simulink model "uz_pmsm_model_2022b"  (R2022b)
settings: Solver=FixedStepAuto  StartTime=0.0  StopTime=0.05  RelTol=1e-3
PreLoadFcn:
  | uz_pmsm_model_init_parameter
PostLoadFcn:
  | % Import the data from Excel for a lookup table
  | FluxMapData = readtable('C:\Users\Philipp\ultrazohm\ultrazohm_sw\ip_cores\uz_pmsm_model\FluxMapData_2023-05-26_13-07-57.csv');
  | % Row indices for lookup table
  | d_current_in_d_axis = FluxMapData(8:27,1:end);
  | % Column indices for lookup table
  | q_current_in_d_axis = FluxMapData(29:48,1:end);
  | % Output values for lookup table
  | d_Flux_d_axis = FluxMapData(50:69,1:end);
values from neighbouring files (symbols this model uses):
  ad1 = ad_1(1)    [LUT_approx_methode2a.m]    (also in LUT_approx_methode2a_clean.m = ad_self(1); LUT_approx_methode_2a_FEM.m; fitting_parameter.mat = 0.03048394862; fitting_parameter_48V_SynRM.mat = 0.0218446789236)
  ad2 = ad_1(2)    [LUT_approx_methode2a.m]    (also in LUT_approx_methode2a_clean.m = ad_self(2); LUT_approx_methode_2a_FEM.m; fitting_parameter.mat = 0.0402440194669; fitting_parameter_48V_SynRM.mat = 0.015691946268)
  ad3 = ad_1(3)    [LUT_approx_methode2a.m]    (also in LUT_approx_methode2a_clean.m = ad_self(3); LUT_approx_methode_2a_FEM.m; fitting_parameter.mat = -16.4812001193; fitting_parameter_48V_SynRM.mat = 2.77465564774)
  ad4 = ad_3_6(1)    [LUT_approx_methode2a.m]    (also in LUT_approx_methode2a_clean.m = ad_4_6(1); LUT_approx_methode_2a_FEM.m; fitting_parameter.mat = 1.2964378241; fitting_parameter_48V_SynRM.mat = 0.0214529395212)
  ad5 = ad_3_6(2)    [LUT_approx_methode2a.m]    (also in LUT_approx_methode2a_clean.m = ad_4_6(2); LUT_approx_methode_2a_FEM.m; fitting_parameter.mat = 0.000618316734858; fitting_parameter_48V_SynRM.mat = 0.0128514742508)
  ad6 = ad_3_6(3)    [LUT_approx_methode2a.m]    (also in LUT_approx_methode2a_clean.m = ad_4_6(3); LUT_approx_methode_2a_FEM.m; fitting_parameter.mat = -12.2755860444; fitting_parameter_48V_SynRM.mat = 2.54408267654)
  aq1 = aq_1(1)    [LUT_approx_methode2a.m]    (also in LUT_approx_methode2a_clean.m = aq_self(1); LUT_approx_methode_2a_FEM.m; fitting_parameter.mat = 0.0048166705291; fitting_parameter_48V_SynRM.mat = 0.00205546577039)
  aq2 = aq_1(2)    [LUT_approx_methode2a.m]    (also in LUT_approx_methode2a_clean.m = aq_self(2); LUT_approx_methode_2a_FEM.m; fitting_parameter.mat = 0.171595255564; fitting_parameter_48V_SynRM.mat = 0.0602932843871)
  aq3 = aq_1(3)    [LUT_approx_methode2a.m]    (also in LUT_approx_methode2a_clean.m = aq_self(3); LUT_approx_methode_2a_FEM.m; fitting_parameter.mat = 0.000926293864031; fitting_parameter_48V_SynRM.mat = 4.42738872822e-05)
  aq4 = aq_3_6(1)    [LUT_approx_methode2a.m]    (also in LUT_approx_methode2a_clean.m = aq_4_6(1); LUT_approx_methode_2a_FEM.m; fitting_parameter.mat = 0.00500187099075; fitting_parameter_48V_SynRM.mat = 0.000698420875152)
  aq5 = aq_3_6(2)    [LUT_approx_methode2a.m]    (also in LUT_approx_methode2a_clean.m = aq_4_6(2); LUT_approx_methode_2a_FEM.m; fitting_parameter.mat = 0.17052123489; fitting_parameter_48V_SynRM.mat = 0.0493122483219)
  aq6 = aq_3_6(3)    [LUT_approx_methode2a.m]    (also in LUT_approx_methode2a_clean.m = aq_4_6(3); LUT_approx_methode_2a_FEM.m; fitting_parameter.mat = 0.00091860845; fitting_parameter_48V_SynRM.mat = 4.14644316065e-05)
  d_current_d_Flux = FluxMapData{1,1:20}    [uz_pmsm_model_init_parameter.m]
  d_current_q_Flux = FluxMapData{66,1:20}    [uz_pmsm_model_init_parameter.m]
  entkopplung_dynamic = false    [compare_simulation_to_measurement.m]    (also in uz_pmsm_model_init_parameter.m; uz_pmsm_model_init_parameter_clean.m)
  entkopplung_linear = true    [compare_simulation_to_measurement.m]    (also in uz_pmsm_model_init_parameter.m; uz_pmsm_model_init_parameter_clean.m = false)
  entkopplung_static = false    [compare_simulation_to_measurement.m]    (also in uz_pmsm_model_init_parameter.m; uz_pmsm_model_init_parameter_clean.m)
  Fid1_Giq1 = ((1/2).*(aq3-aq6).*((q_current_set).^2))+((aq1./aq2).*log(cosh(aq2.*q_current_set)))-((aq4/aq5).*log(cosh(aq5.*q_current_set)))    [LUT_approx_methode2a.m]    (also in LUT_approx_methode2a_clean.m; LUT_approx_methode_2a_FEM.m = (1/2).*(aq3-aq6).*((q_current_set).^2)+((aq1./aq2).*log(cosh; fitting_parameter.mat = -0.00135679401385; fitting_parameter_48V_SynRM.mat = 0.221350145237)
  Fid2_Giq2 = ((ad1./ad2).*(log(cosh(ad2.*(d_current_set-ad3))))) - ((ad4./ad5).*(log(cosh(ad5.*(d_current_set-ad6)))))    [LUT_approx_methode2a.m]    (also in LUT_approx_methode2a_clean.m; LUT_approx_methode_2a_FEM.m = ((ad1./ad2).*(log(cosh(ad2.*(d_current_set-ad3))))) - (((ad1; fitting_parameter.mat = 0.0788137932988; fitting_parameter_48V_SynRM.mat = 0.221214979406)
  Flux_d = FluxMapData{43:62,1:20}'*(1e-3)    [uz_pmsm_model_init_parameter.m]
  Flux_q = FluxMapData{108:127,1:20}'*(1e-3)    [uz_pmsm_model_init_parameter.m]
  friction_coefficient = 0.001    [uz_pmsm_model_init_parameter.m]    (also in uz_pmsm_model_init_parameter_clean.m)
  inertia = 0.000084    (= 8.4e-05)    [uz_pmsm_model_init_parameter.m]    (also in uz_pmsm_model_init_parameter_clean.m)
  L_d = 0.00045    [uz_pmsm_model_init_parameter.m]    (also in uz_pmsm_model_init_parameter_clean.m)
  L_q = 0.002    [uz_pmsm_model_init_parameter.m]    (also in uz_pmsm_model_init_parameter_clean.m)
  parameter_nachfuerung = false    [compare_simulation_to_measurement.m]    (also in uz_pmsm_model_init_parameter.m; uz_pmsm_model_init_parameter_clean.m)
  polepair = 4    [uz_pmsm_model_init_parameter.m]    (also in uz_pmsm_model_init_parameter_clean.m)
  praediktion_entkopplung_nonlinear = false    [compare_simulation_to_measurement.m]    (also in uz_pmsm_model_init_parameter.m; uz_pmsm_model_init_parameter_clean.m = true)
  psi_pm = 0.0194    [uz_pmsm_model_init_parameter.m]    (also in uz_pmsm_model_init_parameter_clean.m)
  q_current_d_Flux = FluxMapData{22:41,1}    [uz_pmsm_model_init_parameter.m]
  q_current_q_Flux = FluxMapData{87:106,1}    [uz_pmsm_model_init_parameter.m]
  R_1 = 0.3    [uz_pmsm_model_init_parameter.m]    (also in uz_pmsm_model_init_parameter_clean.m)
  simulate_mechanical = true    [compare_simulation_to_measurement.m]    (also in export_csv.m = false; uz_pmsm_model_init_parameter.m = false; uz_pmsm_model_init_parameter_clean.m = false)
  simulate_nonlinear_modell = false    [compare_simulation_to_measurement.m]    (also in uz_pmsm_model_init_parameter.m = true; uz_pmsm_model_init_parameter_clean.m = true)
  simulate_open_loop = true    [compare_simulation_to_measurement.m]    (also in export_csv.m; uz_pmsm_model_init_parameter.m = false; uz_pmsm_model_init_parameter_clean.m = false)
  static_friction_torque = 0.01    [uz_pmsm_model_init_parameter.m]    (also in uz_pmsm_model_init_parameter_clean.m)
  tau_sum = 2*ts_regler    (= 0.0001)    [uz_pmsm_model_init_parameter.m]    (also in uz_pmsm_model_init_parameter_clean.m = 8e-05)
  ts = logs{k}.Values    [export_csv.m]    (also in uz_pmsm_model_init_parameter.m = 2e-06; uz_pmsm_model_init_parameter_clean.m = 2e-06)
  ts_regler = 1/20e3    (= 5e-05)    [uz_pmsm_model_init_parameter.m]    (also in uz_pmsm_model_init_parameter_clean.m = 4e-05)
undefined symbols (not defined in the file or in its folder): Ki_Bo_d, Ki_Bo_q, Kp_Bo_d, Kp_Bo_q, Ldq
libraries: slpidlib x6
(part 1 of 4)
settings Model: DataTypeOverride=Off  NumberOfSteps=100  Creator=ts  LastModifiedBy=Philipp
settings SolverCC: AlgebraicLoopSolver=TrustRegion  AutoInsertRateTranBlk=on
settings DataIOCC: LimitDataPoints=on  SaveOutput=off  SaveTime=off
settings OptimizationCC: BlockReduction=off  ConditionallyExecuteInputs=off  DefaultParameterBehavior=Inlined  DefaultUnderspecifiedDataType=single  ReuseModelBlockBuffer=on  LifeSpan=inf
settings DebuggingCC: AlgebraicLoopMsg=error  SingleTaskRateTransMsg=error  UnconnectedInputMsg=warning  UnconnectedOutputMsg=warning  UnconnectedLineMsg=warning  AllowSymbolicDim=off  StrictBusMsg=ErrorOnBusTreatedAsVector  SFUnexpectedBacktrackingDiag=warning  SFNoUnconditionalDefaultTransitionDiag=warning  SFExecutionAtInitializationDiag=none  ArithmeticOperatorsInVariantConditions=warning
settings HardwareCC: ProdBitPerPointer=32  ProdBitPerSizeT=32  ProdBitPerPtrDiffT=32  ProdLargestAtomicFloat=None  ProdIntDivRoundTo=Undefined  ProdEndianess=Unspecified  ProdWordSize=32  ProdHWDeviceType=ASIC/FPGA->ASIC/FPGA  ProdEqTarget=off
settings ModelReferenceCC: EnableRefExpFcnMdlSchedulingChecks=on
settings SFSimCC: SimUseLocalCustomCode=off  CustomCodeUndefinedFunction=UseInterfaceOnly
settings RTWCC: RTWUseLocalCustomCode=off  DLArmComputeVersion=19.05
settings CodeAppCC: StateflowObjectComments=on
settings GRTTargetCC: TargetLangStandard=C89/C90 (ANSI)
settings ConfigComp: CovScope=ReferencedModels  CovMetricSettings=dw  CovSaveCumulativeToWorkspaceVar=on  CovSaveSingleToWorkspaceVar=on  CovExternalEMLEnable=off  CovSFcnEnable=off

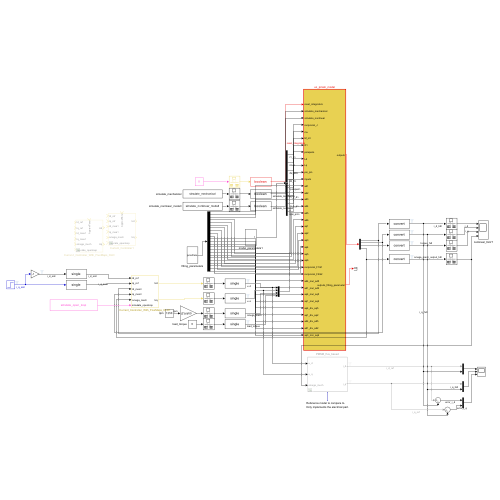
[thumbnail: Simulink's stored preview of the top-level diagram]
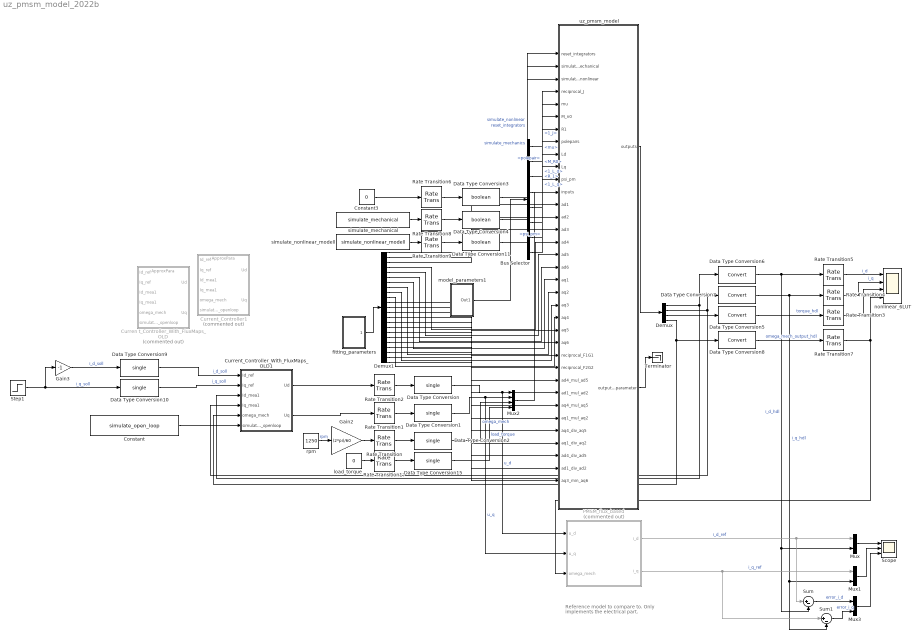
== system uz_pmsm_model_2022b ==
  note: Reference model to compare to.
      | Only implements the electrical part.
  Bus Selector : BusSelector  OutputSignals=1_J,mu,M_R0,R_1,polepair,1_L_d,1_L_q,psi_pm
  Constant : Constant  Value=simulate_open_loop
  Constant3 : Constant  Value=0
  Curren t_Controller_With_FluxMaps_OLD : Subsystem  Commented=on
      settings: PortSchema="{\"entries\":[{\"content\":{\"sides\":[{\"content\":{\"connectorIds\":[\"In1\",\"In2\",\"In3\",\"In4\",\"In5\",\"In6\"]},\"type\":\"ConnectorPlacement.EquallySpacedRectSide\",\"uuid\":\"af970c43-a604-4c86-9598-367deed13f4b\"},{\"content\":{\"connectorIds\":[\"Out1\",\"Out2\"],\"side\":\"RIGHT\"},\"type\":\"ConnectorPlacement.EquallySpacedRectSide\",\"uuid\":\"dab3805d-2102-4aac-8fbd-bf5dcc1227bc\"},{\"content\":{\"connectorIds\":[\"In7\"],\"side\":\"TOP\"},\"type\":\"ConnectorPlacement.EquallySpacedRectSide\",\"uuid\":\"2748ff21-16e6-4765-af5f-5654ece797e9\"}]},\"type\":\"ConnectorPlacement.EquallySpacedConnector\",\"uuid\":\"76312914-9df7-46a3-b8a6-6bdd22bb9fc1\"}],\"packageUris\":[\"http://schema.mathworks.com/mf0/Connector/R2020b\"],\"version\":\"1.0\"}"
  Current_Controller1 : Subsystem  Commented=on
      settings: PortSchema="{\"entries\":[{\"content\":{\"sides\":[{\"content\":{\"connectorIds\":[\"In1\",\"In2\",\"In3\",\"In4\",\"In5\",\"In6\"]},\"type\":\"ConnectorPlacement.EquallySpacedRectSide\",\"uuid\":\"af970c43-a604-4c86-9598-367deed13f4b\"},{\"content\":{\"connectorIds\":[\"Out1\",\"Out2\"],\"side\":\"RIGHT\"},\"type\":\"ConnectorPlacement.EquallySpacedRectSide\",\"uuid\":\"dab3805d-2102-4aac-8fbd-bf5dcc1227bc\"},{\"content\":{\"connectorIds\":[\"In7\"],\"side\":\"TOP\"},\"type\":\"ConnectorPlacement.EquallySpacedRectSide\",\"uuid\":\"2748ff21-16e6-4765-af5f-5654ece797e9\"}]},\"type\":\"ConnectorPlacement.EquallySpacedConnector\",\"uuid\":\"76312914-9df7-46a3-b8a6-6bdd22bb9fc1\"}],\"packageUris\":[\"http://schema.mathworks.com/mf0/Connector/R2020b\"],\"version\":\"1.0\"}"
  Current_Controller_With_FluxMaps_OLD1 : Subsystem
  Data Type Conversion{,1..2,9..10,15} (6 alike) : DataTypeConversion  OutDataTypeStr=single  SaturateOnIntegerOverflow=off  RndMeth=Floor
  Data Type Conversion11 : DataTypeConversion  OutDataTypeStr=boolean  SaturateOnIntegerOverflow=off  RndMeth=Floor
  Data Type Conversion3 : DataTypeConversion  OutDataTypeStr=boolean  SaturateOnIntegerOverflow=off  RndMeth=Floor
  Data Type Conversion4 : DataTypeConversion  OutDataTypeStr=boolean  SaturateOnIntegerOverflow=off  RndMeth=Floor
  Data Type Conversion{5..8} (4 alike) : DataTypeConversion  SaturateOnIntegerOverflow=off  RndMeth=Floor
  Demux : Demux
  Demux1 : Demux  Outputs=23
  Gain2 : Gain  Gain=(2*pi)/60
  Gain3 : Gain  Gain=-1
  Mux : Mux  Inputs=2
  Mux1 : Mux  Inputs=2
  Mux2 : Mux
  Mux3 : Mux  Inputs=2
  PMSM_flux_based : Subsystem  Commented=on
  Rate Transition{,1..2,6,8..9,17} (7 alike) : RateTransition  OutPortSampleTime=ts
  Rate Transition{3..5,7} (4 alike) : RateTransition
  Scope : Scope  NumInputPorts=3
  Step1 : Step  Time=0.025  After=10
  Sum : Sum  Inputs=|+-
  Sum1 : Sum  Inputs=|+-
  Terminator : Terminator
  fitting_parameters : Subsystem
  load_torque : Constant  Value=0
  model_parameters1 : Subsystem
  nonlinear_6LUT : Scope  NumInputPorts=4
  rpm : Constant  Value=1250
  simulate_mechanical : Constant  Value=simulate_mechanical
  simulate_nonlinear_modell : Constant  Value=simulate_nonlinear_modell
  uz_pmsm_model : Subsystem  TreatAsAtomicUnit=on
  wires:
  Rate Transition/1 -> Data Type Conversion2/1
  Rate Transition1/1 -> Data Type Conversion1/1
  Rate Transition2/1 -> Data Type Conversion/1
  Data Type Conversion6/1 -> Mux/2, Sum/2, Rate Transition5/1  "i_d_hdl"
  Data Type Conversion7/1 -> Rate Transition4/1, Mux1/2, Sum1/2  "i_q_hdl"
  Data Type Conversion5/1 -> Rate Transition3/1  "torque_hdl"
  Rate Transition4/1 -> nonlinear_6LUT/2  "i_q"
  Rate Transition5/1 -> nonlinear_6LUT/1  "i_d"
  Rate Transition3/1 -> nonlinear_6LUT/3
  Rate Transition6/1 -> Data Type Conversion3/1
  Constant3/1 -> Rate Transition6/1
  Rate Transition8/1 -> Data Type Conversion4/1
  simulate_mechanical/1 -> Rate Transition8/1
  Data Type Conversion3/1 -> uz_pmsm_model/1(reset_integrators)  "reset_integrators"
  Data Type Conversion4/1 -> uz_pmsm_model/2(simulate_mechanical)  "simulate_mechanics"
  load_torque/1 -> Rate Transition17/1
  Rate Transition17/1 -> Data Type Conversion15/1
  Mux/1 -> Scope/1
  Mux1/1 -> Scope/2
  PMSM_flux_based/2(i_q) -> Mux1/1, Sum1/1  "i_q_ref"
  PMSM_flux_based/1(i_d) -> Mux/1, Sum/1  "i_d_ref"
  Data Type Conversion8/1 -> Rate Transition7/1  "omega_mech_output_hdl"
  Rate Transition7/1 -> PMSM_flux_based/3(omega_mech), nonlinear_6LUT/4
  Bus Selector/1 -> uz_pmsm_model/4(reciprocal_J)  "<1_J>"
  Bus Selector/2 -> uz_pmsm_model/5(mu)  "<mu>"
  Bus Selector/3 -> uz_pmsm_model/6(M_n0)  "<M_R0>"
  Bus Selector/4 -> uz_pmsm_model/7(R1)  "<R_1>"
  Bus Selector/5 -> uz_pmsm_model/8(polepairs)  "<polepair>"
  model_parameters1/1(Out1) -> Bus Selector/1
  Sum/1 -> Mux3/1  "error_i_d"
  Sum1/1 -> Mux3/2  "error_i_q"
  Mux3/1 -> Scope/3
  Step1/1 -> Gain3/1, Data Type Conversion10/1  "i_q_soll"
  Demux/3 -> Data Type Conversion5/1
  Gain3/1 -> Data Type Conversion9/1  "i_d_soll"
  Demux/1 -> Current_Controller_With_FluxMaps_OLD1/3(Id_mea1), Data Type Conversion6/1
  Demux/4 -> Current_Controller_With_FluxMaps_OLD1/5(omega_mech), Data Type Conversion8/1
  Demux/2 -> Data Type Conversion7/1, Current_Controller_With_FluxMaps_OLD1/4(Iq_mea1)
  Data Type Conversion/1 -> PMSM_flux_based/1(u_d), Mux2/1  "u_d"
  Data Type Conversion1/1 -> PMSM_flux_based/2(u_q), Mux2/2  "u_q"
  Data Type Conversion15/1 -> Mux2/4  "load_torque"
  Data Type Conversion2/1 -> Mux2/3  "omega_mech"
  Mux2/1 -> uz_pmsm_model/12(inputs)
  uz_pmsm_model/1(outputs) -> Demux/1
  Data Type Conversion9/1 -> Current_Controller_With_FluxMaps_OLD1/1(Id_ref)  "i_d_soll"
  Data Type Conversion10/1 -> Current_Controller_With_FluxMaps_OLD1/2(Iq_ref)  "i_q_soll"
  Current_Controller_With_FluxMaps_OLD1/1(Ud) -> Rate Transition2/1
  Current_Controller_With_FluxMaps_OLD1/2(Uq) -> Rate Transition1/1
  Gain2/1 -> Rate Transition/1
  Constant/1 -> Current_Controller_With_FluxMaps_OLD1/6(simulate_openloop)
  rpm/1 -> Gain2/1  "rpm"
  simulate_nonlinear_modell/1 -> Rate Transition9/1
  Rate Transition9/1 -> Data Type Conversion11/1
  Bus Selector/6 -> uz_pmsm_model/9(Ld)  "<1_L_d>"
  Bus Selector/7 -> uz_pmsm_model/10(Lq)  "<1_L_q>"
  Bus Selector/8 -> uz_pmsm_model/11(psi_pm)  "<psi_pm>"
  Data Type Conversion11/1 -> uz_pmsm_model/3(simulate_nonlinear)  "simulate_nonlinear"
  fitting_parameters/1(ApproxPara) -> Demux1/1
  Demux1/1 -> uz_pmsm_model/13(ad1)
  Demux1/2 -> uz_pmsm_model/14(ad2)
  Demux1/3 -> uz_pmsm_model/15(ad3)
  Demux1/4 -> uz_pmsm_model/16(ad4)
  Demux1/5 -> uz_pmsm_model/17(ad5)
  Demux1/6 -> uz_pmsm_model/18(ad6)
  Demux1/7 -> uz_pmsm_model/19(aq1)
  Demux1/8 -> uz_pmsm_model/20(aq2)
  Demux1/9 -> uz_pmsm_model/21(aq3)
  Demux1/10 -> uz_pmsm_model/22(aq4)
  Demux1/11 -> uz_pmsm_model/23(aq5)
  Demux1/12 -> uz_pmsm_model/24(aq6)
  Demux1/13 -> uz_pmsm_model/25(reciprocal_F1G1)
  Demux1/14 -> uz_pmsm_model/26(reciprocal_F2G2)
  Demux1/15 -> uz_pmsm_model/27(ad4_mul_ad5)
  Demux1/16 -> uz_pmsm_model/28(ad1_mul_ad2)
  Demux1/17 -> uz_pmsm_model/29(aq4_mul_aq5)
  Demux1/18 -> uz_pmsm_model/30(aq1_mul_aq2)
  Demux1/19 -> uz_pmsm_model/31(aq4_div_aq5)
  Demux1/20 -> uz_pmsm_model/32(aq1_div_aq2)
  Demux1/21 -> uz_pmsm_model/33(ad4_div_ad5)
  Demux1/22 -> uz_pmsm_model/34(ad1_div_ad2)
  Demux1/23 -> uz_pmsm_model/35(aq3_min_aq6)
  uz_pmsm_model/2(outputs_fitting_parameter) -> Terminator/1

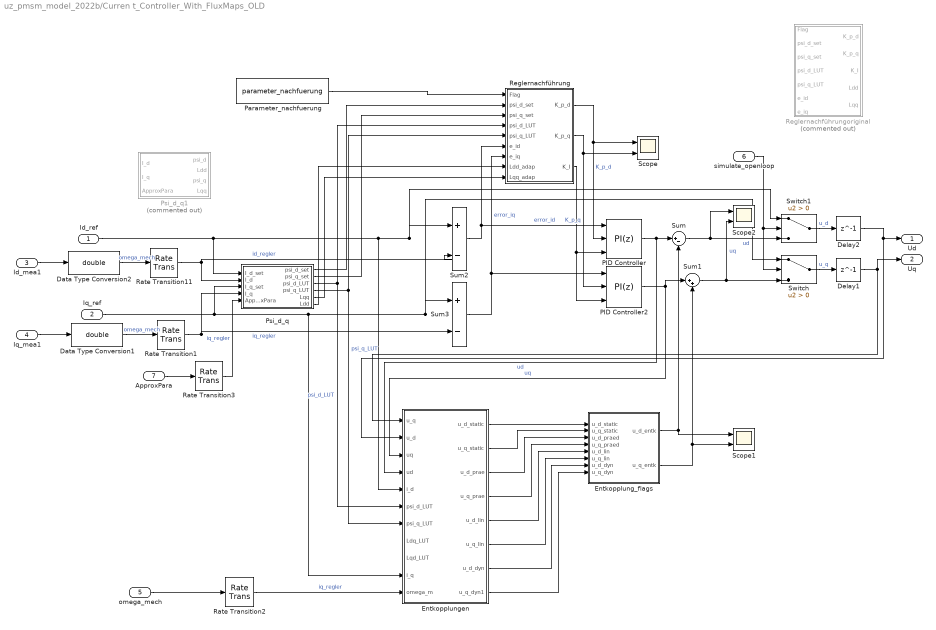
== system uz_pmsm_model_2022b/Curren t_Controller_With_FluxMaps_OLD ==
  Id_ref : Inport
  Iq_ref : Inport  Port=2
  Id_mea1 : Inport  Port=3
  Iq_mea1 : Inport  Port=4
  omega_mech : Inport  Port=5
  simulate_openloop : Inport  Port=6
  ApproxPara : Inport  Port=7
  Data Type Conversion1 : DataTypeConversion  OutDataTypeStr=double  SaturateOnIntegerOverflow=off  RndMeth=Floor
  Data Type Conversion2 : DataTypeConversion  OutDataTypeStr=double  SaturateOnIntegerOverflow=off  RndMeth=Floor
  Delay1 : Delay  DelayLength=1
  Delay2 : Delay  DelayLength=1
  Entkopplung_flags : Subsystem
  Entkopplungen : Subsystem
  PID Controller : slpidlib/PID Controller  Controller=PI  Form=Parallel  TimeDomain=Discrete-time  UseExternalTs=off  SampleTime=-1  IntegratorMethod=Forward Euler  FilterMethod=Forward Euler  ControllerParametersSource=external  P=Kp_Bo_d  I=Ki_Bo_d  UseKiTs=off  D=0  N=100  UseFilter=on  TunerSelectOption=Transfer Function Based (PID Tuner App)  InitialConditionSource=internal  InitialConditionForIntegrator=0  InitialConditionForFilter=0  DifferentiatorICPrevScaledInput=0  ExternalReset=none  TrackingMode=off  Kt=1  LimitOutput=off  SatLimitsSource=internal  UpperSaturationLimit=48  LowerSaturationLimit=-48  LinearizeAsGain=off  AntiWindupMode=clamping  Kb=1  LimitIntegrator=off  UpperIntegratorSaturationLimit=48  LowerIntegratorSaturationLimit=-48  POutMin=[]  POutMax=[]  IOutMin=[]  IOutMax=[]  DOutMin=[]  DOutMax=[]  NOutMin=[]  NOutMax=[]  SumOutMin=[]  SumOutMax=[]  SaturationOutMin=[]  SaturationOutMax=[]  PParamMin=[]  PParamMax=[]  IParamMin=[]  IParamMax=[]  DParamMin=[]  DParamMax=[]  NParamMin=[]  NParamMax=[]  KbParamMin=[]  KbParamMax=[]  KtParamMin=[]  KtParamMax=[]  KbOutMin=[]  KbOutMax=[]  KtOutMin=[]  KtOutMax=[]  IntegratorOutMin=[]  IntegratorOutMax=[]  FilterOutMin=[]  FilterOutMax=[]  SumI1OutMin=[]  SumI1OutMax=[]  SumI2OutMin=[]  SumI2OutMax=[]  SumI3OutMin=[]  SumI3OutMax=[]  SumI4OutMin=[]  SumI4OutMax=[]  SumDOutMin=[]  SumDOutMax=[]  DifferentiatorOutMin=[]  DifferentiatorOutMax=[]  FilterDiffOutCoefMin=[]  FilterDiffOutCoefMax=[]  ReciprocalOutMin=[]  ReciprocalOutMax=[]  SumDenOutMin=[]  SumDenOutMax=[]  SumNumOutMin=[]  SumNumOutMax=[]  DivideOutMin=[]  DivideOutMax=[]  UdiffTsProdOutMin=[]  UdiffTsProdOutMax=[]  NTsProdOutMin=[]  NTsProdOutMax=[]  UintegralTsProdOutMin=[]  UintegralTsProdOutMax=[]  UngainTsProdOutMin=[]  UngainTsProdOutMax=[]  IntegratorContinuousStateAttributes=''  IntegratorStateMustResolveToSignalObject=off  IntegratorRTWStateStorageClass=Auto  FilterContinuousStateAttributes=''  FilterStateMustResolveToSignalObject=off  FilterRTWStateStorageClass=Auto  ParallelPVariant=ExternalParameters  IdealPVariant=Disabled  IVariant=ExternalParameters  DVariant=Disabled  IntegratorVariant=Discrete  SatVariant=Disabled  AWVariant=Passthrough  PCopyVariant=Disabled  TRVariant=Disabled  FdbkBlocksVariant=Forward  IdealPFdbkVariant=Disabled  SatFdbkVariant=Disabled  DerivativeFilterVariant=Disabled  NVariant=Disabled  NCopyVariant=Disabled_SignalSpec  FilterICVariant=Disabled  IntegratorICVariant=InternalICs  ExternalResetVariant=Disabled  TRSumVariant=Passthrough  SumFdbkVariant=Disabled  SumVariant=Sum_PI  TsampFilterVariant=InternalTs  TsampNgainVariant=Passthrough  TsampIntegralVariant=Disabled_SignalSpec  ExternalSaturationOutDataTypeStr=Inherit: Same as second input
  PID Controller2 : slpidlib/PID Controller  Controller=PI  Form=Parallel  TimeDomain=Discrete-time  UseExternalTs=off  SampleTime=-1  IntegratorMethod=Forward Euler  FilterMethod=Forward Euler  ControllerParametersSource=external  P=Kp_Bo_q  I=Ki_Bo_q  UseKiTs=off  D=0  N=100  UseFilter=on  TunerSelectOption=Transfer Function Based (PID Tuner App)  InitialConditionSource=internal  InitialConditionForIntegrator=0  InitialConditionForFilter=0  DifferentiatorICPrevScaledInput=0  ExternalReset=none  TrackingMode=off  Kt=1  LimitOutput=off  SatLimitsSource=internal  UpperSaturationLimit=48  LowerSaturationLimit=-48  LinearizeAsGain=off  AntiWindupMode=clamping  Kb=1  LimitIntegrator=off  UpperIntegratorSaturationLimit=48  LowerIntegratorSaturationLimit=-48  POutMin=[]  POutMax=[]  IOutMin=[]  IOutMax=[]  DOutMin=[]  DOutMax=[]  NOutMin=[]  NOutMax=[]  SumOutMin=[]  SumOutMax=[]  SaturationOutMin=[]  SaturationOutMax=[]  PParamMin=[]  PParamMax=[]  IParamMin=[]  IParamMax=[]  DParamMin=[]  DParamMax=[]  NParamMin=[]  NParamMax=[]  KbParamMin=[]  KbParamMax=[]  KtParamMin=[]  KtParamMax=[]  KbOutMin=[]  KbOutMax=[]  KtOutMin=[]  KtOutMax=[]  IntegratorOutMin=[]  IntegratorOutMax=[]  FilterOutMin=[]  FilterOutMax=[]  SumI1OutMin=[]  SumI1OutMax=[]  SumI2OutMin=[]  SumI2OutMax=[]  SumI3OutMin=[]  SumI3OutMax=[]  SumI4OutMin=[]  SumI4OutMax=[]  SumDOutMin=[]  SumDOutMax=[]  DifferentiatorOutMin=[]  DifferentiatorOutMax=[]  FilterDiffOutCoefMin=[]  FilterDiffOutCoefMax=[]  ReciprocalOutMin=[]  ReciprocalOutMax=[]  SumDenOutMin=[]  SumDenOutMax=[]  SumNumOutMin=[]  SumNumOutMax=[]  DivideOutMin=[]  DivideOutMax=[]  UdiffTsProdOutMin=[]  UdiffTsProdOutMax=[]  NTsProdOutMin=[]  NTsProdOutMax=[]  UintegralTsProdOutMin=[]  UintegralTsProdOutMax=[]  UngainTsProdOutMin=[]  UngainTsProdOutMax=[]  IntegratorContinuousStateAttributes=''  IntegratorStateMustResolveToSignalObject=off  IntegratorRTWStateStorageClass=Auto  FilterContinuousStateAttributes=''  FilterStateMustResolveToSignalObject=off  FilterRTWStateStorageClass=Auto  ParallelPVariant=ExternalParameters  IdealPVariant=Disabled  IVariant=ExternalParameters  DVariant=Disabled  IntegratorVariant=Discrete  SatVariant=Disabled  AWVariant=Passthrough  PCopyVariant=Disabled  TRVariant=Disabled  FdbkBlocksVariant=Forward  IdealPFdbkVariant=Disabled  SatFdbkVariant=Disabled  DerivativeFilterVariant=Disabled  NVariant=Disabled  NCopyVariant=Disabled_SignalSpec  FilterICVariant=Disabled  IntegratorICVariant=InternalICs  ExternalResetVariant=Disabled  TRSumVariant=Passthrough  SumFdbkVariant=Disabled  SumVariant=Sum_PI  TsampFilterVariant=InternalTs  TsampNgainVariant=Passthrough  TsampIntegralVariant=Disabled_SignalSpec  ExternalSaturationOutDataTypeStr=Inherit: Same as second input
  Parameter_nachfuerung : Constant  Value=parameter_nachfuerung
  Psi_d_q : Subsystem
  Psi_d_q1 : Subsystem  Commented=on
  Rate Transition{1..3,11} (4 alike) : RateTransition  OutPortSampleTime=ts_regler
  Reglernachführung : Subsystem
  Reglernachführungoriginal : Subsystem  Commented=on
  Scope : Scope  NumInputPorts=2
  Scope1 : Scope  NumInputPorts=2
  Scope2 : Scope  NumInputPorts=2
  Sum : Sum  Inputs=|+-
  Sum1 : Sum  Inputs=|++
  Sum2 : Sum  Inputs=|+-
  Sum3 : Sum  Inputs=|+-
  Switch : Switch  Criteria=u2 > Threshold  SaturateOnIntegerOverflow=off  InputSameDT=off
  Switch1 : Switch  Criteria=u2 > Threshold  SaturateOnIntegerOverflow=off  InputSameDT=off
  Ud : Outport
  Uq : Outport  Port=2
  wires:
  Sum3/1 -> Reglernachführung/7(e_iq), PID Controller2/1  "error_iq"
  Sum2/1 -> PID Controller/1, Reglernachführung/6(e_id)  "error_id"
  Sum/1 -> Scope2/1, Switch1/3  "ud"
  PID Controller/1 -> Entkopplungen/4(ud), Sum/1  "ud"
  PID Controller2/1 -> Sum1/1, Entkopplungen/3(uq)  "uq"
  Sum1/1 -> Scope2/2, Switch/3  "uq"
  Iq_ref/1 -> Entkopplungen/10(i_q), Sum3/1, Switch/1, Psi_d_q/3(I_q_set)
  Id_ref/1 -> Psi_d_q/1(I_d_set), Entkopplungen/5(i_d), Sum2/1, Switch1/1
  Switch/1 -> Delay1/1  "u_q"
  Switch1/1 -> Delay2/1  "u_d"
  simulate_openloop/1 -> Switch/2, Switch1/2
  Reglernachführung/1(K_p_d) -> PID Controller/2, Scope/1  "K_p_d"
  Reglernachführung/2(K_p_q) -> PID Controller2/2, Scope/2  "K_p_q"
  Reglernachführung/3(K_I) -> PID Controller2/3, PID Controller/3
  Id_mea1/1 -> Data Type Conversion2/1
  Iq_mea1/1 -> Data Type Conversion1/1
  Psi_d_q/3(psi_d_LUT) -> Entkopplungen/6(psi_d_LUT), Reglernachführung/4(psi_d_LUT)  "psi_d_LUT"
  Psi_d_q/4(psi_q_LUT) -> Entkopplungen/7(psi_q_LUT), Reglernachführung/5(psi_q_LUT)  "psi_q_LUT"
  Parameter_nachfuerung/1 -> Reglernachführung/1(Flag)
  Psi_d_q/1(psi_d_set) -> Reglernachführung/2(psi_d_set)
  Psi_d_q/2(psi_q_set) -> Reglernachführung/3(psi_q_set)
  omega_mech/1 -> Rate Transition2/1
  Entkopplungen/1(u_d_static) -> Entkopplung_flags/1(u_d_static)
  Entkopplungen/2(u_q_static) -> Entkopplung_flags/2(u_q_static)
  Entkopplungen/3(u_d_prae) -> Entkopplung_flags/3(u_d_praed)
  Entkopplungen/4(u_q_prae) -> Entkopplung_flags/4(u_q_praed)
  Entkopplungen/5(u_d_lin) -> Entkopplung_flags/5(u_d_lin)
  Entkopplungen/6(u_q_lin) -> Entkopplung_flags/6(u_q_lin)
  Entkopplung_flags/1(u_d_entk) -> Scope1/1, Sum/2
  Entkopplung_flags/2(u_q_entk) -> Scope1/2, Sum1/2
  Rate Transition11/1 -> Sum2/2, Psi_d_q/2(I_d)  "id_regler"
  Rate Transition1/1 -> Sum3/2, Psi_d_q/4(I_q)  "iq_regler"
  Rate Transition2/1 -> Entkopplungen/11(omega_m)  "iq_regler"
  Delay2/1 -> Ud/1, Entkopplungen/2(u_d)
  Delay1/1 -> Uq/1, Entkopplungen/1(u_q)
  Entkopplungen/7(u_d_dyn) -> Entkopplung_flags/7(u_d_dyn)
  Entkopplungen/8(u_q_dyn1) -> Entkopplung_flags/8(u_q_dyn)
  ApproxPara/1 -> Rate Transition3/1
  Rate Transition3/1 -> Psi_d_q/5(ApproxPara)  "iq_regler"
  Data Type Conversion2/1 -> Rate Transition11/1  "omega_mech"
  Data Type Conversion1/1 -> Rate Transition1/1  "omega_mech"
  Psi_d_q/5(Lqq) -> Reglernachführung/9(Lqq_adap)
  Psi_d_q/6(Ldd) -> Reglernachführung/8(Ldd_adap)

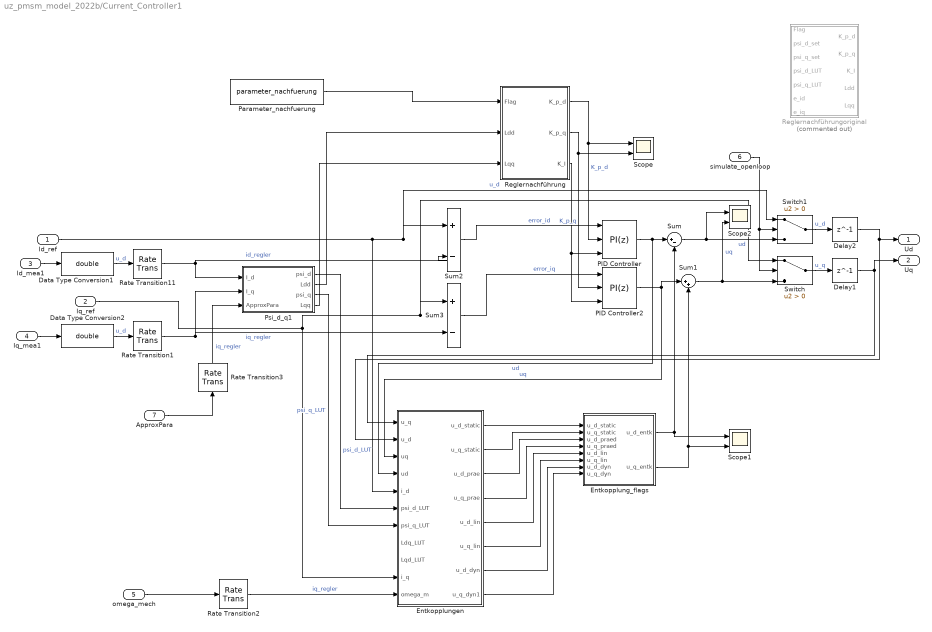
== system uz_pmsm_model_2022b/Current_Controller1 ==
  Id_ref : Inport
  Iq_ref : Inport  Port=2
  Id_mea1 : Inport  Port=3
  Iq_mea1 : Inport  Port=4
  omega_mech : Inport  Port=5
  simulate_openloop : Inport  Port=6
  ApproxPara : Inport  Port=7
  Data Type Conversion1 : DataTypeConversion  OutDataTypeStr=double  SaturateOnIntegerOverflow=off  RndMeth=Floor
  Data Type Conversion2 : DataTypeConversion  OutDataTypeStr=double  SaturateOnIntegerOverflow=off  RndMeth=Floor
  Delay1 : Delay  DelayLength=1
  Delay2 : Delay  DelayLength=1
  Entkopplung_flags : Subsystem
  Entkopplungen : Subsystem
  PID Controller : slpidlib/PID Controller  Controller=PI  Form=Parallel  TimeDomain=Discrete-time  UseExternalTs=off  SampleTime=-1  IntegratorMethod=Forward Euler  FilterMethod=Forward Euler  ControllerParametersSource=external  P=Kp_Bo_d  I=Ki_Bo_d  UseKiTs=off  D=0  N=100  UseFilter=on  TunerSelectOption=Transfer Function Based (PID Tuner App)  InitialConditionSource=internal  InitialConditionForIntegrator=0  InitialConditionForFilter=0  DifferentiatorICPrevScaledInput=0  ExternalReset=none  TrackingMode=off  Kt=1  LimitOutput=off  SatLimitsSource=internal  UpperSaturationLimit=48  LowerSaturationLimit=-48  LinearizeAsGain=off  AntiWindupMode=clamping  Kb=1  LimitIntegrator=off  UpperIntegratorSaturationLimit=48  LowerIntegratorSaturationLimit=-48  POutMin=[]  POutMax=[]  IOutMin=[]  IOutMax=[]  DOutMin=[]  DOutMax=[]  NOutMin=[]  NOutMax=[]  SumOutMin=[]  SumOutMax=[]  SaturationOutMin=[]  SaturationOutMax=[]  PParamMin=[]  PParamMax=[]  IParamMin=[]  IParamMax=[]  DParamMin=[]  DParamMax=[]  NParamMin=[]  NParamMax=[]  KbParamMin=[]  KbParamMax=[]  KtParamMin=[]  KtParamMax=[]  KbOutMin=[]  KbOutMax=[]  KtOutMin=[]  KtOutMax=[]  IntegratorOutMin=[]  IntegratorOutMax=[]  FilterOutMin=[]  FilterOutMax=[]  SumI1OutMin=[]  SumI1OutMax=[]  SumI2OutMin=[]  SumI2OutMax=[]  SumI3OutMin=[]  SumI3OutMax=[]  SumI4OutMin=[]  SumI4OutMax=[]  SumDOutMin=[]  SumDOutMax=[]  DifferentiatorOutMin=[]  DifferentiatorOutMax=[]  FilterDiffOutCoefMin=[]  FilterDiffOutCoefMax=[]  ReciprocalOutMin=[]  ReciprocalOutMax=[]  SumDenOutMin=[]  SumDenOutMax=[]  SumNumOutMin=[]  SumNumOutMax=[]  DivideOutMin=[]  DivideOutMax=[]  UdiffTsProdOutMin=[]  UdiffTsProdOutMax=[]  NTsProdOutMin=[]  NTsProdOutMax=[]  UintegralTsProdOutMin=[]  UintegralTsProdOutMax=[]  UngainTsProdOutMin=[]  UngainTsProdOutMax=[]  IntegratorContinuousStateAttributes=''  IntegratorStateMustResolveToSignalObject=off  IntegratorRTWStateStorageClass=Auto  FilterContinuousStateAttributes=''  FilterStateMustResolveToSignalObject=off  FilterRTWStateStorageClass=Auto  ParallelPVariant=ExternalParameters  IdealPVariant=Disabled  IVariant=ExternalParameters  DVariant=Disabled  IntegratorVariant=Discrete  SatVariant=Disabled  AWVariant=Passthrough  PCopyVariant=Disabled  TRVariant=Disabled  FdbkBlocksVariant=Forward  IdealPFdbkVariant=Disabled  SatFdbkVariant=Disabled  DerivativeFilterVariant=Disabled  NVariant=Disabled  NCopyVariant=Disabled_SignalSpec  FilterICVariant=Disabled  IntegratorICVariant=InternalICs  ExternalResetVariant=Disabled  TRSumVariant=Passthrough  SumFdbkVariant=Disabled  SumVariant=Sum_PI  TsampFilterVariant=InternalTs  TsampNgainVariant=Passthrough  TsampIntegralVariant=Disabled_SignalSpec  ExternalSaturationOutDataTypeStr=Inherit: Same as second input
  PID Controller2 : slpidlib/PID Controller  Controller=PI  Form=Parallel  TimeDomain=Discrete-time  UseExternalTs=off  SampleTime=-1  IntegratorMethod=Forward Euler  FilterMethod=Forward Euler  ControllerParametersSource=external  P=Kp_Bo_q  I=Ki_Bo_q  UseKiTs=off  D=0  N=100  UseFilter=on  TunerSelectOption=Transfer Function Based (PID Tuner App)  InitialConditionSource=internal  InitialConditionForIntegrator=0  InitialConditionForFilter=0  DifferentiatorICPrevScaledInput=0  ExternalReset=none  TrackingMode=off  Kt=1  LimitOutput=off  SatLimitsSource=internal  UpperSaturationLimit=48  LowerSaturationLimit=-48  LinearizeAsGain=off  AntiWindupMode=clamping  Kb=1  LimitIntegrator=off  UpperIntegratorSaturationLimit=48  LowerIntegratorSaturationLimit=-48  POutMin=[]  POutMax=[]  IOutMin=[]  IOutMax=[]  DOutMin=[]  DOutMax=[]  NOutMin=[]  NOutMax=[]  SumOutMin=[]  SumOutMax=[]  SaturationOutMin=[]  SaturationOutMax=[]  PParamMin=[]  PParamMax=[]  IParamMin=[]  IParamMax=[]  DParamMin=[]  DParamMax=[]  NParamMin=[]  NParamMax=[]  KbParamMin=[]  KbParamMax=[]  KtParamMin=[]  KtParamMax=[]  KbOutMin=[]  KbOutMax=[]  KtOutMin=[]  KtOutMax=[]  IntegratorOutMin=[]  IntegratorOutMax=[]  FilterOutMin=[]  FilterOutMax=[]  SumI1OutMin=[]  SumI1OutMax=[]  SumI2OutMin=[]  SumI2OutMax=[]  SumI3OutMin=[]  SumI3OutMax=[]  SumI4OutMin=[]  SumI4OutMax=[]  SumDOutMin=[]  SumDOutMax=[]  DifferentiatorOutMin=[]  DifferentiatorOutMax=[]  FilterDiffOutCoefMin=[]  FilterDiffOutCoefMax=[]  ReciprocalOutMin=[]  ReciprocalOutMax=[]  SumDenOutMin=[]  SumDenOutMax=[]  SumNumOutMin=[]  SumNumOutMax=[]  DivideOutMin=[]  DivideOutMax=[]  UdiffTsProdOutMin=[]  UdiffTsProdOutMax=[]  NTsProdOutMin=[]  NTsProdOutMax=[]  UintegralTsProdOutMin=[]  UintegralTsProdOutMax=[]  UngainTsProdOutMin=[]  UngainTsProdOutMax=[]  IntegratorContinuousStateAttributes=''  IntegratorStateMustResolveToSignalObject=off  IntegratorRTWStateStorageClass=Auto  FilterContinuousStateAttributes=''  FilterStateMustResolveToSignalObject=off  FilterRTWStateStorageClass=Auto  ParallelPVariant=ExternalParameters  IdealPVariant=Disabled  IVariant=ExternalParameters  DVariant=Disabled  IntegratorVariant=Discrete  SatVariant=Disabled  AWVariant=Passthrough  PCopyVariant=Disabled  TRVariant=Disabled  FdbkBlocksVariant=Forward  IdealPFdbkVariant=Disabled  SatFdbkVariant=Disabled  DerivativeFilterVariant=Disabled  NVariant=Disabled  NCopyVariant=Disabled_SignalSpec  FilterICVariant=Disabled  IntegratorICVariant=InternalICs  ExternalResetVariant=Disabled  TRSumVariant=Passthrough  SumFdbkVariant=Disabled  SumVariant=Sum_PI  TsampFilterVariant=InternalTs  TsampNgainVariant=Passthrough  TsampIntegralVariant=Disabled_SignalSpec  ExternalSaturationOutDataTypeStr=Inherit: Same as second input
  Parameter_nachfuerung : Constant  Value=parameter_nachfuerung
  Psi_d_q1 : Subsystem
  Rate Transition{1..3,11} (4 alike) : RateTransition  OutPortSampleTime=ts_regler
  Reglernachführung : Subsystem
  Reglernachführungoriginal : Subsystem  Commented=on
  Scope : Scope  NumInputPorts=2
  Scope1 : Scope  NumInputPorts=2
  Scope2 : Scope  NumInputPorts=2
  Sum : Sum  Inputs=|+-
  Sum1 : Sum  Inputs=|++
  Sum2 : Sum  Inputs=|+-
  Sum3 : Sum  Inputs=|+-
  Switch : Switch  Criteria=u2 > Threshold  SaturateOnIntegerOverflow=off  InputSameDT=off
  Switch1 : Switch  Criteria=u2 > Threshold  SaturateOnIntegerOverflow=off  InputSameDT=off
  Ud : Outport
  Uq : Outport  Port=2
  wires:
  Sum3/1 -> PID Controller2/1  "error_iq"
  Sum2/1 -> PID Controller/1  "error_id"
  Sum/1 -> Scope2/1, Switch1/3  "ud"
  PID Controller/1 -> Entkopplungen/4(ud), Sum/1  "ud"
  PID Controller2/1 -> Sum1/1, Entkopplungen/3(uq)  "uq"
  Sum1/1 -> Scope2/2, Switch/3  "uq"
  Iq_ref/1 -> Sum3/1, Switch/1, Entkopplungen/10(i_q)
  Switch/1 -> Delay1/1  "u_q"
  Switch1/1 -> Delay2/1  "u_d"
  simulate_openloop/1 -> Switch/2, Switch1/2
  Reglernachführung/1(K_p_d) -> PID Controller/2, Scope/1  "K_p_d"
  Reglernachführung/2(K_p_q) -> PID Controller2/2, Scope/2  "K_p_q"
  Reglernachführung/3(K_I) -> PID Controller2/3, PID Controller/3
  Id_mea1/1 -> Data Type Conversion1/1
  Iq_mea1/1 -> Data Type Conversion2/1
  Psi_d_q1/1(psi_d) -> Entkopplungen/6(psi_d_LUT)  "psi_d_LUT"
  Psi_d_q1/3(psi_q) -> Entkopplungen/7(psi_q_LUT)  "psi_q_LUT"
  Parameter_nachfuerung/1 -> Reglernachführung/1(Flag)
  omega_mech/1 -> Rate Transition2/1
  Entkopplungen/1(u_d_static) -> Entkopplung_flags/1(u_d_static)
  Entkopplungen/2(u_q_static) -> Entkopplung_flags/2(u_q_static)
  Entkopplungen/3(u_d_prae) -> Entkopplung_flags/3(u_d_praed)
  Entkopplungen/4(u_q_prae) -> Entkopplung_flags/4(u_q_praed)
  Entkopplungen/5(u_d_lin) -> Entkopplung_flags/5(u_d_lin)
  Entkopplungen/6(u_q_lin) -> Entkopplung_flags/6(u_q_lin)
  Entkopplung_flags/1(u_d_entk) -> Scope1/1, Sum/2
  Entkopplung_flags/2(u_q_entk) -> Scope1/2, Sum1/2
  Rate Transition11/1 -> Sum2/2, Psi_d_q1/1(I_d)  "id_regler"
  Rate Transition1/1 -> Psi_d_q1/2(I_q), Sum3/2  "iq_regler"
  Rate Transition2/1 -> Entkopplungen/11(omega_m)  "iq_regler"
  Delay2/1 -> Ud/1, Entkopplungen/2(u_d)
  Delay1/1 -> Uq/1, Entkopplungen/1(u_q)
  Entkopplungen/7(u_d_dyn) -> Entkopplung_flags/7(u_d_dyn)
  Entkopplungen/8(u_q_dyn1) -> Entkopplung_flags/8(u_q_dyn)
  Psi_d_q1/2(Ldd) -> Reglernachführung/2(Ldd)
  Psi_d_q1/4(Lqq) -> Reglernachführung/3(Lqq)
  ApproxPara/1 -> Rate Transition3/1
  Rate Transition3/1 -> Psi_d_q1/3(ApproxPara)  "iq_regler"
  Id_ref/1 -> Entkopplungen/5(i_d), Sum2/1, Switch1/1  "u_d"
  Data Type Conversion1/1 -> Rate Transition11/1  "u_d"
  Data Type Conversion2/1 -> Rate Transition1/1  "u_d"

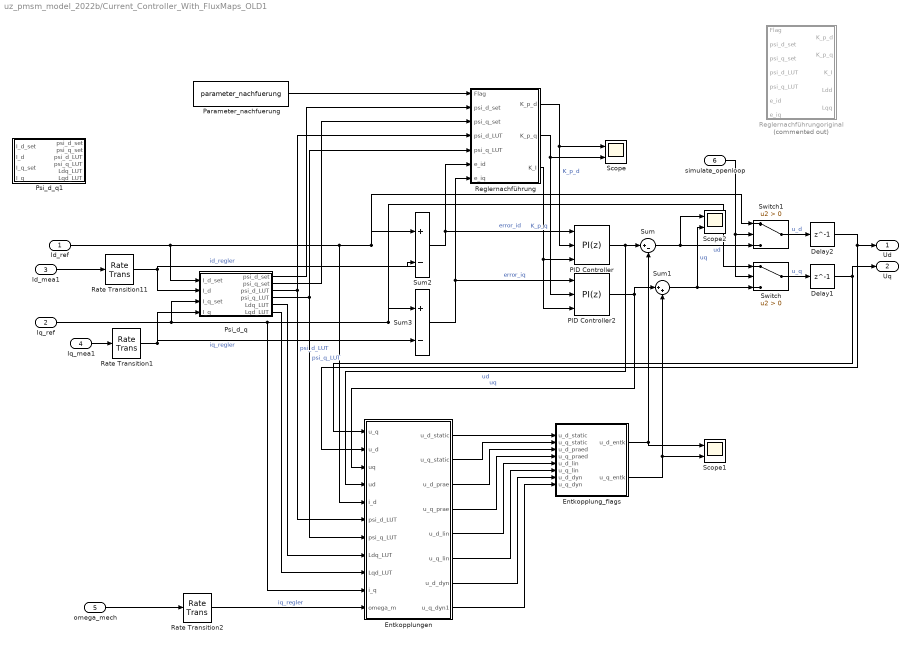
== system uz_pmsm_model_2022b/Current_Controller_With_FluxMaps_OLD1 ==
  Id_ref : Inport
  Iq_ref : Inport  Port=2
  Id_mea1 : Inport  Port=3
  Iq_mea1 : Inport  Port=4
  omega_mech : Inport  Port=5
  simulate_openloop : Inport  Port=6
  Delay1 : Delay  DelayLength=1
  Delay2 : Delay  DelayLength=1
  Entkopplung_flags : Subsystem
  Entkopplungen : Subsystem
  PID Controller : slpidlib/PID Controller  Controller=PI  Form=Parallel  TimeDomain=Discrete-time  UseExternalTs=off  SampleTime=-1  IntegratorMethod=Forward Euler  FilterMethod=Forward Euler  ControllerParametersSource=external  P=Kp_Bo_d  I=Ki_Bo_d  UseKiTs=off  D=0  N=100  UseFilter=on  TunerSelectOption=Transfer Function Based (PID Tuner App)  InitialConditionSource=internal  InitialConditionForIntegrator=0  InitialConditionForFilter=0  DifferentiatorICPrevScaledInput=0  ExternalReset=none  TrackingMode=off  Kt=1  LimitOutput=off  SatLimitsSource=internal  UpperSaturationLimit=48  LowerSaturationLimit=-48  LinearizeAsGain=off  AntiWindupMode=clamping  Kb=1  LimitIntegrator=off  UpperIntegratorSaturationLimit=48  LowerIntegratorSaturationLimit=-48  POutMin=[]  POutMax=[]  IOutMin=[]  IOutMax=[]  DOutMin=[]  DOutMax=[]  NOutMin=[]  NOutMax=[]  SumOutMin=[]  SumOutMax=[]  SaturationOutMin=[]  SaturationOutMax=[]  PParamMin=[]  PParamMax=[]  IParamMin=[]  IParamMax=[]  DParamMin=[]  DParamMax=[]  NParamMin=[]  NParamMax=[]  KbParamMin=[]  KbParamMax=[]  KtParamMin=[]  KtParamMax=[]  KbOutMin=[]  KbOutMax=[]  KtOutMin=[]  KtOutMax=[]  IntegratorOutMin=[]  IntegratorOutMax=[]  FilterOutMin=[]  FilterOutMax=[]  SumI1OutMin=[]  SumI1OutMax=[]  SumI2OutMin=[]  SumI2OutMax=[]  SumI3OutMin=[]  SumI3OutMax=[]  SumI4OutMin=[]  SumI4OutMax=[]  SumDOutMin=[]  SumDOutMax=[]  DifferentiatorOutMin=[]  DifferentiatorOutMax=[]  FilterDiffOutCoefMin=[]  FilterDiffOutCoefMax=[]  ReciprocalOutMin=[]  ReciprocalOutMax=[]  SumDenOutMin=[]  SumDenOutMax=[]  SumNumOutMin=[]  SumNumOutMax=[]  DivideOutMin=[]  DivideOutMax=[]  UdiffTsProdOutMin=[]  UdiffTsProdOutMax=[]  NTsProdOutMin=[]  NTsProdOutMax=[]  UintegralTsProdOutMin=[]  UintegralTsProdOutMax=[]  UngainTsProdOutMin=[]  UngainTsProdOutMax=[]  IntegratorContinuousStateAttributes=''  IntegratorStateMustResolveToSignalObject=off  IntegratorRTWStateStorageClass=Auto  FilterContinuousStateAttributes=''  FilterStateMustResolveToSignalObject=off  FilterRTWStateStorageClass=Auto  ParallelPVariant=ExternalParameters  IdealPVariant=Disabled  IVariant=ExternalParameters  DVariant=Disabled  IntegratorVariant=Discrete  SatVariant=Disabled  AWVariant=Passthrough  PCopyVariant=Disabled  TRVariant=Disabled  FdbkBlocksVariant=Forward  IdealPFdbkVariant=Disabled  SatFdbkVariant=Disabled  DerivativeFilterVariant=Disabled  NVariant=Disabled  NCopyVariant=Disabled_SignalSpec  FilterICVariant=Disabled  IntegratorICVariant=InternalICs  ExternalResetVariant=Disabled  TRSumVariant=Passthrough  SumFdbkVariant=Disabled  SumVariant=Sum_PI  TsampFilterVariant=InternalTs  TsampNgainVariant=Passthrough  TsampIntegralVariant=Disabled_SignalSpec  ExternalSaturationOutDataTypeStr=Inherit: Same as second input
  PID Controller2 : slpidlib/PID Controller  Controller=PI  Form=Parallel  TimeDomain=Discrete-time  UseExternalTs=off  SampleTime=-1  IntegratorMethod=Forward Euler  FilterMethod=Forward Euler  ControllerParametersSource=external  P=Kp_Bo_q  I=Ki_Bo_q  UseKiTs=off  D=0  N=100  UseFilter=on  TunerSelectOption=Transfer Function Based (PID Tuner App)  InitialConditionSource=internal  InitialConditionForIntegrator=0  InitialConditionForFilter=0  DifferentiatorICPrevScaledInput=0  ExternalReset=none  TrackingMode=off  Kt=1  LimitOutput=off  SatLimitsSource=internal  UpperSaturationLimit=48  LowerSaturationLimit=-48  LinearizeAsGain=off  AntiWindupMode=clamping  Kb=1  LimitIntegrator=off  UpperIntegratorSaturationLimit=48  LowerIntegratorSaturationLimit=-48  POutMin=[]  POutMax=[]  IOutMin=[]  IOutMax=[]  DOutMin=[]  DOutMax=[]  NOutMin=[]  NOutMax=[]  SumOutMin=[]  SumOutMax=[]  SaturationOutMin=[]  SaturationOutMax=[]  PParamMin=[]  PParamMax=[]  IParamMin=[]  IParamMax=[]  DParamMin=[]  DParamMax=[]  NParamMin=[]  NParamMax=[]  KbParamMin=[]  KbParamMax=[]  KtParamMin=[]  KtParamMax=[]  KbOutMin=[]  KbOutMax=[]  KtOutMin=[]  KtOutMax=[]  IntegratorOutMin=[]  IntegratorOutMax=[]  FilterOutMin=[]  FilterOutMax=[]  SumI1OutMin=[]  SumI1OutMax=[]  SumI2OutMin=[]  SumI2OutMax=[]  SumI3OutMin=[]  SumI3OutMax=[]  SumI4OutMin=[]  SumI4OutMax=[]  SumDOutMin=[]  SumDOutMax=[]  DifferentiatorOutMin=[]  DifferentiatorOutMax=[]  FilterDiffOutCoefMin=[]  FilterDiffOutCoefMax=[]  ReciprocalOutMin=[]  ReciprocalOutMax=[]  SumDenOutMin=[]  SumDenOutMax=[]  SumNumOutMin=[]  SumNumOutMax=[]  DivideOutMin=[]  DivideOutMax=[]  UdiffTsProdOutMin=[]  UdiffTsProdOutMax=[]  NTsProdOutMin=[]  NTsProdOutMax=[]  UintegralTsProdOutMin=[]  UintegralTsProdOutMax=[]  UngainTsProdOutMin=[]  UngainTsProdOutMax=[]  IntegratorContinuousStateAttributes=''  IntegratorStateMustResolveToSignalObject=off  IntegratorRTWStateStorageClass=Auto  FilterContinuousStateAttributes=''  FilterStateMustResolveToSignalObject=off  FilterRTWStateStorageClass=Auto  ParallelPVariant=ExternalParameters  IdealPVariant=Disabled  IVariant=ExternalParameters  DVariant=Disabled  IntegratorVariant=Discrete  SatVariant=Disabled  AWVariant=Passthrough  PCopyVariant=Disabled  TRVariant=Disabled  FdbkBlocksVariant=Forward  IdealPFdbkVariant=Disabled  SatFdbkVariant=Disabled  DerivativeFilterVariant=Disabled  NVariant=Disabled  NCopyVariant=Disabled_SignalSpec  FilterICVariant=Disabled  IntegratorICVariant=InternalICs  ExternalResetVariant=Disabled  TRSumVariant=Passthrough  SumFdbkVariant=Disabled  SumVariant=Sum_PI  TsampFilterVariant=InternalTs  TsampNgainVariant=Passthrough  TsampIntegralVariant=Disabled_SignalSpec  ExternalSaturationOutDataTypeStr=Inherit: Same as second input
  Parameter_nachfuerung : Constant  Value=parameter_nachfuerung
  Psi_d_q : Subsystem
  Psi_d_q1 : Subsystem
  Rate Transition1 : RateTransition  OutPortSampleTime=ts_regler
  Rate Transition11 : RateTransition  OutPortSampleTime=ts_regler
  Rate Transition2 : RateTransition  OutPortSampleTime=ts_regler
  Reglernachführung : Subsystem
  Reglernachführungoriginal : Subsystem  Commented=on
  Scope : Scope  NumInputPorts=2
  Scope1 : Scope  NumInputPorts=2
  Scope2 : Scope  NumInputPorts=2
  Sum : Sum  Inputs=|+-
  Sum1 : Sum  Inputs=|++
  Sum2 : Sum  Inputs=|+-
  Sum3 : Sum  Inputs=|+-
  Switch : Switch  Criteria=u2 > Threshold  SaturateOnIntegerOverflow=off  InputSameDT=off
  Switch1 : Switch  Criteria=u2 > Threshold  SaturateOnIntegerOverflow=off  InputSameDT=off
  Ud : Outport
  Uq : Outport  Port=2
  wires:
  Sum3/1 -> Reglernachführung/7(e_iq), PID Controller2/1  "error_iq"
  Sum2/1 -> PID Controller/1, Reglernachführung/6(e_id)  "error_id"
  Sum/1 -> Scope2/1, Switch1/3  "ud"
  PID Controller/1 -> Entkopplungen/4(ud), Sum/1  "ud"
  PID Controller2/1 -> Sum1/1, Entkopplungen/3(uq)  "uq"
  Sum1/1 -> Scope2/2, Switch/3  "uq"
  Iq_ref/1 -> Entkopplungen/10(i_q), Sum3/1, Switch/1, Psi_d_q/3(I_q_set)
  Id_ref/1 -> Psi_d_q/1(I_d_set), Entkopplungen/5(i_d), Sum2/1, Switch1/1
  Switch/1 -> Delay1/1  "u_q"
  Switch1/1 -> Delay2/1  "u_d"
  simulate_openloop/1 -> Switch/2, Switch1/2
  Reglernachführung/1(K_p_d) -> PID Controller/2, Scope/1  "K_p_d"
  Reglernachführung/2(K_p_q) -> PID Controller2/2, Scope/2  "K_p_q"
  Reglernachführung/3(K_I) -> PID Controller2/3, PID Controller/3
  Id_mea1/1 -> Rate Transition11/1
  Iq_mea1/1 -> Rate Transition1/1
  Psi_d_q/3(psi_d_LUT) -> Entkopplungen/6(psi_d_LUT), Reglernachführung/4(psi_d_LUT)  "psi_d_LUT"
  Psi_d_q/4(psi_q_LUT) -> Entkopplungen/7(psi_q_LUT), Reglernachführung/5(psi_q_LUT)  "psi_q_LUT"
  Parameter_nachfuerung/1 -> Reglernachführung/1(Flag)
  Psi_d_q/1(psi_d_set) -> Reglernachführung/2(psi_d_set)
  Psi_d_q/2(psi_q_set) -> Reglernachführung/3(psi_q_set)
  omega_mech/1 -> Rate Transition2/1
  Entkopplungen/1(u_d_static) -> Entkopplung_flags/1(u_d_static)
  Entkopplungen/2(u_q_static) -> Entkopplung_flags/2(u_q_static)
  Entkopplungen/3(u_d_prae) -> Entkopplung_flags/3(u_d_praed)
  Entkopplungen/4(u_q_prae) -> Entkopplung_flags/4(u_q_praed)
  Entkopplungen/5(u_d_lin) -> Entkopplung_flags/5(u_d_lin)
  Entkopplungen/6(u_q_lin) -> Entkopplung_flags/6(u_q_lin)
  Entkopplung_flags/1(u_d_entk) -> Scope1/1, Sum/2
  Entkopplung_flags/2(u_q_entk) -> Scope1/2, Sum1/2
  Rate Transition11/1 -> Sum2/2, Psi_d_q/2(I_d)  "id_regler"
  Rate Transition1/1 -> Sum3/2, Psi_d_q/4(I_q)  "iq_regler"
  Rate Transition2/1 -> Entkopplungen/11(omega_m)  "iq_regler"
  Delay2/1 -> Ud/1, Entkopplungen/2(u_d)
  Delay1/1 -> Uq/1, Entkopplungen/1(u_q)
  Entkopplungen/7(u_d_dyn) -> Entkopplung_flags/7(u_d_dyn)
  Entkopplungen/8(u_q_dyn1) -> Entkopplung_flags/8(u_q_dyn)
  Psi_d_q/5(Ldq_LUT) -> Entkopplungen/8(Ldq_LUT)
  Psi_d_q/6(Lqd_LUT) -> Entkopplungen/9(Lqd_LUT)

== system uz_pmsm_model_2022b/PMSM_flux_based ==
  u_d : Inport
  u_q : Inport  Port=2
  omega_mech : Inport  Port=3
  Constant : Constant  Value=psi_pm
  Gain : Gain  Gain=R_1
  Gain1 : Gain  Gain=1/L_d
  Gain2 : Gain  Gain=R_1
  Gain3 : Gain  Gain=1/L_q
  Gain6 : Gain  Gain=polepair
  Integrator : Integrator
  Integrator1 : Integrator
  Product : Product
  Product1 : Product
  Sum : Sum  Inputs=-++
  Sum1 : Sum  Inputs=-+-
  Sum2 : Sum  Inputs=+-
  i_d : Outport
  i_q : Outport  Port=2
  wires:
  u_d/1 -> Sum/2
  u_q/1 -> Sum1/2
  Sum/1 -> Integrator/1
  Gain/1 -> Sum/1
  Integrator/1 -> Product1/2, Sum2/1
  Constant/1 -> Sum2/2
  Sum2/1 -> Gain1/1
  Gain1/1 -> Gain/1, i_d/1
  Gain6/1 -> Product1/1, Product/1
  Product/1 -> Sum/3
  Integrator1/1 -> Gain3/1, Product/2
  Product1/1 -> Sum1/3
  Sum1/1 -> Integrator1/1
  Gain2/1 -> Sum1/1
  Gain3/1 -> i_q/1, Gain2/1
  omega_mech/1 -> Gain6/1

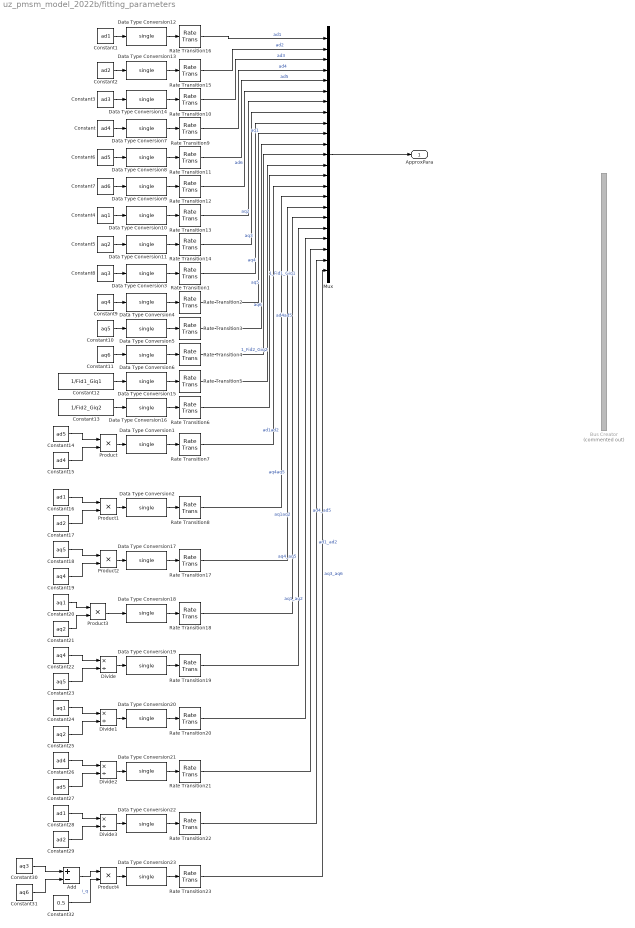
== system uz_pmsm_model_2022b/fitting_parameters ==
  Add : Sum  Inputs=+-
  Bus Creator : BusCreator  Commented=on  Inputs=23
  Constant : Constant  Value=ad4
  Constant1 : Constant  Value=ad1
  Constant10 : Constant  Value=aq5
  Constant11 : Constant  Value=aq6
  Constant12 : Constant  Value=1/Fid1_Giq1
  Constant13 : Constant  Value=1/Fid2_Giq2
  Constant14 : Constant  Value=ad5
  Constant15 : Constant  Value=ad4
  Constant16 : Constant  Value=ad1
  Constant17 : Constant  Value=ad2
  Constant18 : Constant  Value=aq5
  Constant19 : Constant  Value=aq4
  Constant2 : Constant  Value=ad2
  Constant20 : Constant  Value=aq1
  Constant21 : Constant  Value=aq2
  Constant22 : Constant  Value=aq4
  Constant23 : Constant  Value=aq5
  Constant24 : Constant  Value=aq1
  Constant25 : Constant  Value=aq2
  Constant26 : Constant  Value=ad4
  Constant27 : Constant  Value=ad5
  Constant28 : Constant  Value=ad1
  Constant29 : Constant  Value=ad2
  Constant3 : Constant  Value=ad3
  Constant30 : Constant  Value=aq3
  Constant31 : Constant  Value=aq6
  Constant32 : Constant  Value=0.5  OutDataTypeStr=double  SampleTime=-1
  Constant4 : Constant  Value=aq1
  Constant5 : Constant  Value=aq2
  Constant6 : Constant  Value=ad5
  Constant7 : Constant  Value=ad6
  Constant8 : Constant  Value=aq3
  Constant9 : Constant  Value=aq4
  Data Type Conversion{1..23} (23 alike) : DataTypeConversion  OutDataTypeStr=single  SaturateOnIntegerOverflow=off  RndMeth=Floor
  Divide{,1..3} (4 alike) : Product  Inputs=*/
  Mux : Mux  Inputs=23
  Product{,1..4} (5 alike) : Product
  Rate Transition{1..23} (23 alike) : RateTransition  OutPortSampleTime=ts
  ApproxPara : Outport
  wires:
  Constant1/1 -> Data Type Conversion12/1
  Constant/1 -> Data Type Conversion7/1
  Rate Transition10/1 -> Mux/3  "ad3"
  Rate Transition14/1 -> Mux/8  "aq2"
  Constant3/1 -> Data Type Conversion14/1
  Rate Transition12/1 -> Mux/6  "ad6"
  Rate Transition16/1 -> Mux/1  "ad1"
  Rate Transition13/1 -> Mux/7  "aq1"
  Constant5/1 -> Data Type Conversion11/1
  Constant7/1 -> Data Type Conversion9/1
  Rate Transition15/1 -> Mux/2  "ad2"
  Rate Transition9/1 -> Mux/4  "ad4"
  Constant6/1 -> Data Type Conversion8/1
  Constant4/1 -> Data Type Conversion10/1
  Rate Transition11/1 -> Mux/5  "ad5"
  Constant2/1 -> Data Type Conversion13/1
  Rate Transition1/1 -> Mux/9  "aq3"
  Constant8/1 -> Data Type Conversion3/1
  Rate Transition2/1 -> Mux/10  "aq4"
  Constant9/1 -> Data Type Conversion4/1
  Rate Transition3/1 -> Mux/11  "aq5"
  Constant10/1 -> Data Type Conversion5/1
  Rate Transition4/1 -> Mux/12  "aq6"
  Constant11/1 -> Data Type Conversion6/1
  Rate Transition5/1 -> Mux/13  "1_Fid1_Giq1"
  Constant12/1 -> Data Type Conversion15/1
  Constant13/1 -> Data Type Conversion16/1
  Rate Transition6/1 -> Mux/14  "1_Fid2_Giq2"
  Data Type Conversion11/1 -> Rate Transition14/1
  Data Type Conversion10/1 -> Rate Transition13/1
  Data Type Conversion9/1 -> Rate Transition12/1
  Data Type Conversion12/1 -> Rate Transition16/1
  Data Type Conversion13/1 -> Rate Transition15/1
  Data Type Conversion14/1 -> Rate Transition10/1
  Data Type Conversion7/1 -> Rate Transition9/1
  Data Type Conversion8/1 -> Rate Transition11/1
  Data Type Conversion3/1 -> Rate Transition1/1
  Data Type Conversion4/1 -> Rate Transition2/1
  Data Type Conversion5/1 -> Rate Transition3/1
  Data Type Conversion6/1 -> Rate Transition4/1
  Data Type Conversion15/1 -> Rate Transition5/1
  Data Type Conversion16/1 -> Rate Transition6/1
  Constant14/1 -> Product/1
  Constant15/1 -> Product/2
  Product/1 -> Data Type Conversion1/1
  Data Type Conversion1/1 -> Rate Transition7/1
  Rate Transition7/1 -> Mux/15  "ad4ad5"
  Rate Transition8/1 -> Mux/16  "ad1ad2"
  Constant16/1 -> Product1/1
  Constant17/1 -> Product1/2
  Data Type Conversion2/1 -> Rate Transition8/1
  Product1/1 -> Data Type Conversion2/1
  Constant18/1 -> Product2/1
  Constant19/1 -> Product2/2
  Data Type Conversion17/1 -> Rate Transition17/1
  Product2/1 -> Data Type Conversion17/1
  Rate Transition18/1 -> Mux/18  "aq1aq2"
  Product3/1 -> Data Type Conversion18/1
  Data Type Conversion18/1 -> Rate Transition18/1
  Constant21/1 -> Product3/2
  Constant20/1 -> Product3/1
  Rate Transition17/1 -> Mux/17  "aq4aq5"
  Divide/1 -> Data Type Conversion19/1
  Data Type Conversion19/1 -> Rate Transition19/1
  Constant22/1 -> Divide/1
  Constant23/1 -> Divide/2
  Rate Transition19/1 -> Mux/19  "aq4_aq5"
  Constant24/1 -> Divide1/1
  Constant25/1 -> Divide1/2
  Rate Transition20/1 -> Mux/20  "aq1_aq2"
  Divide1/1 -> Data Type Conversion20/1
  Data Type Conversion20/1 -> Rate Transition20/1
  Data Type Conversion21/1 -> Rate Transition21/1
  Divide2/1 -> Data Type Conversion21/1
  Rate Transition21/1 -> Mux/21  "ad4_ad5"
  Constant27/1 -> Divide2/2
  Constant26/1 -> Divide2/1
  Constant28/1 -> Divide3/1
  Rate Transition22/1 -> Mux/22  "ad1_ad2"
  Constant29/1 -> Divide3/2
  Divide3/1 -> Data Type Conversion22/1
  Data Type Conversion22/1 -> Rate Transition22/1
  Data Type Conversion23/1 -> Rate Transition23/1
  Constant30/1 -> Add/1
  Constant31/1 -> Add/2
  Rate Transition23/1 -> Mux/23  "aq3_aq6"
  Product4/1 -> Data Type Conversion23/1
  Constant32/1 -> Product4/2  "i_q"
  Add/1 -> Product4/1
  Mux/1 -> ApproxPara/1
